simulink model "chuandongmoxing"  (R2014a)
settings: Solver=ode45  StartTime=0.0  StopTime=10.0  RelTol=1e-3
settings Model: Creator=hsinwang  LastModifiedBy=hsinwang

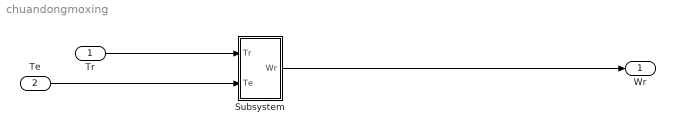
== system chuandongmoxing ==
  Tr : Inport
  Te : Inport  Port=2
  Subsystem : Subsystem
  Wr : Outport
  wires:
  Tr/1 -> Subsystem/1(Tr)
  Te/1 -> Subsystem/2(Te)
  Subsystem/1(Wr) -> Wr/1

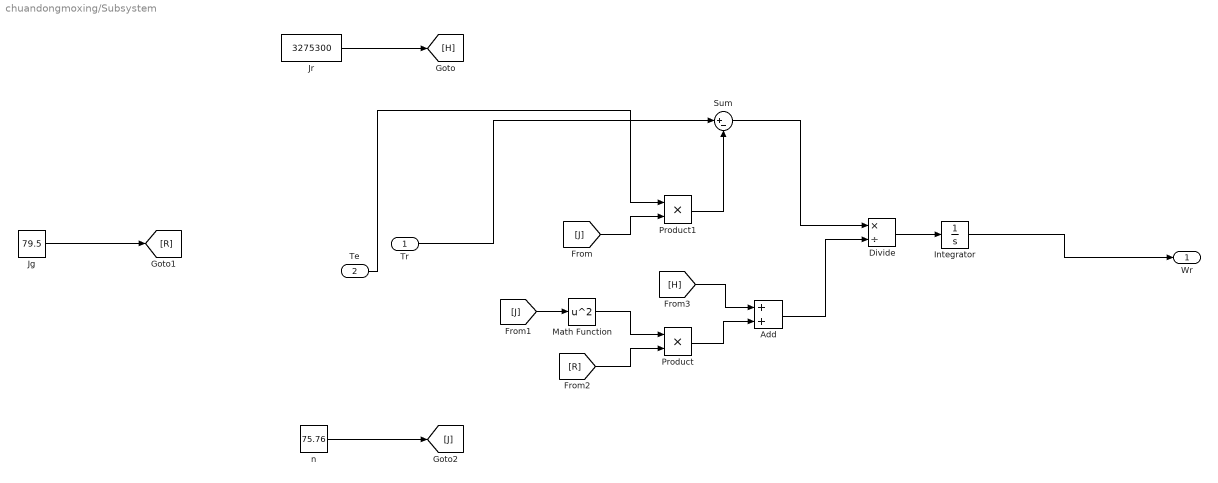
== system chuandongmoxing/Subsystem ==
  Tr : Inport
  Te : Inport  Port=2
  Add : Sum
  Divide : Product  Inputs=*/
  Integrator : Integrator
  "Jg " : Constant  Value=79.5
  "Jr " : Constant  Value=3275300
  Math Function : Math  Operator=square  SaturateOnIntegerOverflow=on
  Product : Product
  Product1 : Product
  Sum : Sum  Inputs=|+-
  n : Constant  Value=75.76
  Wr : Outport
  wires:
  Te/1 -> Product1/1
  [R] -> Product/2
  Product/1 -> Add/2
  "Jr "/1 -> [H]
  Integrator/1 -> Wr/1
  [J] -> Math Function/1
  "Jg "/1 -> [R]
  Tr/1 -> Sum/1
  Math Function/1 -> Product/1
  Divide/1 -> Integrator/1
  Add/1 -> Divide/2
  [J] -> Product1/2
  n/1 -> [J]
  Sum/1 -> Divide/1
  [H] -> Add/1
  Product1/1 -> Sum/2
